simulink model "RollYawDamperController"  (R2021a)
settings: Solver=VariableStepAuto  StartTime=0.0  StopTime=500  RelTol=1e-3
undefined symbols (not defined in the file): A_lat, B_lat, C_lat, D_lat, g, U0
libraries: simulink_extras x3, cstblocks x2
settings Model: Creator=User01  LastModifiedBy=User01

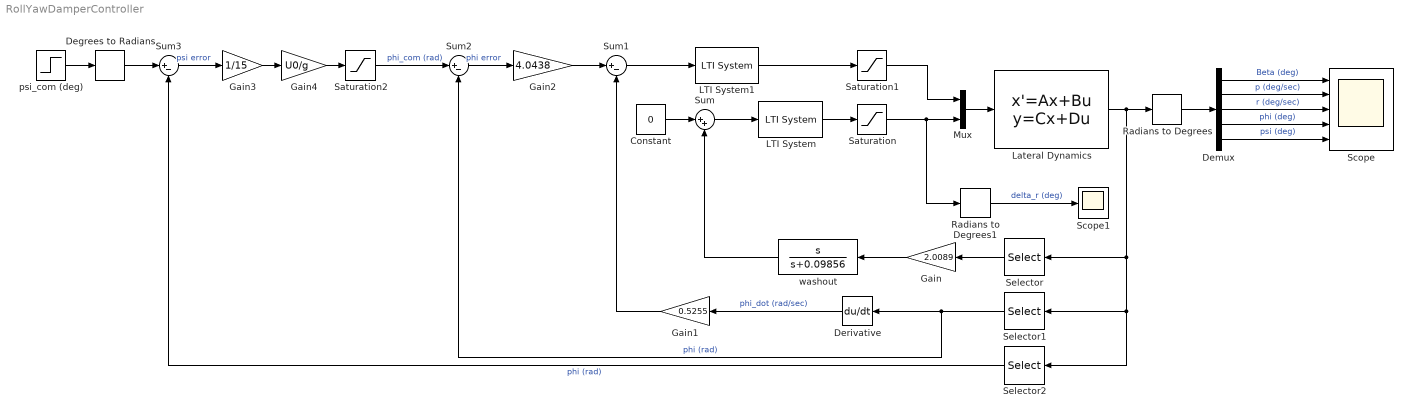
== system RollYawDamperController ==
  Constant : Constant  Value=0
  Degrees to Radians : simulink_extras/Transformations/Degrees to Radians
  Demux : Demux  Outputs=5
  Derivative : Derivative
  Gain : Gain  Gain=2.0089
  Gain1 : Gain  Gain=0.5255
  Gain2 : Gain  Gain=4.0438
  Gain3 : Gain  Gain=1/15
  Gain4 : Gain  Gain=U0/g
  LTI System : cstblocks/LTI System  sys=servo  IC=[]
  LTI System1 : cstblocks/LTI System  sys=servo  IC=[]
  Lateral Dynamics : StateSpace  A=A_lat  B=B_lat  C=C_lat  D=D_lat  InitialCondition=0
  Mux : Mux  Inputs=2
  Radians to Degrees : simulink_extras/Transformations/Radians to Degrees
  Radians to Degrees1 : simulink_extras/Transformations/Radians to Degrees
  Saturation : Saturate  UpperLimit=15*pi/180  LowerLimit=-15*pi/180
  Saturation1 : Saturate  UpperLimit=50*pi/180  LowerLimit=-50*pi/180
  Saturation2 : Saturate  UpperLimit=30*pi/180  LowerLimit=-30*pi/180
  Scope : Scope  NumInputPorts=5
  Scope1 : Scope
  Selector : Selector  InputPortWidth=5  IndexOptions=Index vector (dialog)  Indices=3  OutputSizes=1
  Selector1 : Selector  InputPortWidth=5  IndexOptions=Index vector (dialog)  Indices=4  OutputSizes=1
  Selector2 : Selector  InputPortWidth=5  IndexOptions=Index vector (dialog)  Indices=5  OutputSizes=1
  Sum : Sum  Inputs=|++
  Sum1 : Sum  Inputs=|+-
  Sum2 : Sum  Inputs=|+-
  Sum3 : Sum  Inputs=|+-
  psi_com (deg) : Step  After=360  SampleTime=0
  washout : TransferFcn  Numerator=[1 0]  Denominator=[1 0.09856]
  wires:
  Lateral Dynamics/1 -> Selector2/1, Selector1/1, Selector/1, Radians to Degrees/1
  Mux/1 -> Lateral Dynamics/1
  Saturation/1 -> Mux/2, Radians to Degrees1/1
  LTI System/1 -> Saturation/1
  Sum/1 -> LTI System/1
  Constant/1 -> Sum/1
  Selector/1 -> Gain/1
  washout/1 -> Sum/2
  Demux/1 -> Scope/1  "Beta (deg)"
  Demux/2 -> Scope/2  "p (deg/sec)"
  Demux/3 -> Scope/3  "r (deg/sec)"
  Demux/4 -> Scope/4  "phi (deg)"
  Demux/5 -> Scope/5  "psi (deg)"
  Saturation1/1 -> Mux/1
  Radians to Degrees/1 -> Demux/1
  Radians to Degrees1/1 -> Scope1/1  "delta_r (deg)"
  LTI System1/1 -> Saturation1/1
  Sum1/1 -> LTI System1/1
  Selector1/1 -> Derivative/1, Sum2/2  "phi (rad)"
  Derivative/1 -> Gain1/1  "phi_dot (rad/sec)"
  Gain1/1 -> Sum1/2
  Sum2/1 -> Gain2/1  "phi error"
  Degrees to Radians/1 -> Sum3/1
  Selector2/1 -> Sum3/2  "phi (rad)"
  Gain4/1 -> Saturation2/1
  Gain3/1 -> Gain4/1
  Sum3/1 -> Gain3/1  "psi error"
  Gain2/1 -> Sum1/1
  psi_com (deg)/1 -> Degrees to Radians/1
  Saturation2/1 -> Sum2/1  "phi_com (rad)"
  Gain/1 -> washout/1
